simulink model "Part4_1"  (R2021a)
settings: Solver=VariableStepAuto  StartTime=0.0  StopTime=10.0  RelTol=1e-3
settings Model: Creator=theod  LastModifiedBy=theod

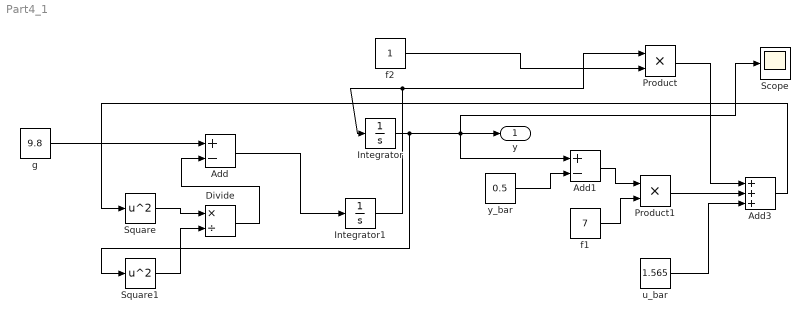
== system Part4_1 ==
  Add : Sum  Inputs=+-
  Add1 : Sum  Inputs=+-
  Add3 : Sum  Inputs=+++
  Divide : Product  Inputs=*/
  Integrator : Integrator  InitialCondition=1.3
  Integrator1 : Integrator  InitialCondition=0.5
  Product : Product
  Product1 : Product
  Scope : Scope
  Square : Math  Operator=square  SaturateOnIntegerOverflow=on
  Square1 : Math  Operator=square  SaturateOnIntegerOverflow=on
  f1 : Constant  Value=7
  f2 : Constant
  g : Constant  Value=9.8
  u_bar : Constant  Value=1.565
  y_bar : Constant  Value=0.5
  y : Outport
  wires:
  Integrator1/1 -> Integrator/1, Product/1
  Integrator/1 -> Square1/1, Scope/1, Add1/1, y/1
  Square/1 -> Divide/1
  Square1/1 -> Divide/2
  Divide/1 -> Add/2
  g/1 -> Add/1
  Add/1 -> Integrator1/1
  f2/1 -> Product/2
  y_bar/1 -> Add1/2
  Add1/1 -> Product1/1
  f1/1 -> Product1/2
  Product1/1 -> Add3/2
  Product/1 -> Add3/1
  u_bar/1 -> Add3/3
  Add3/1 -> Square/1
